simulink model "zad1"  (Simulink 7.7)
settings: Solver=ode45  StartTime=0.0  StopTime=t_sim  RelTol=1e-3
values from neighbouring files (symbols this model uses):
  ICX = -0.2    [zadatak1.m]    (also in zadatak2.m = 2; zadatak4.m = 0.4)
  ICY = -0.6    [zadatak1.m]    (also in zadatak2.m = 4; zadatak4.m = 1)
settings Model: Creator=Domagoj  LastModifiedBy=Domagoj
settings DebuggingCC: SolverPrmCheckMsg=none

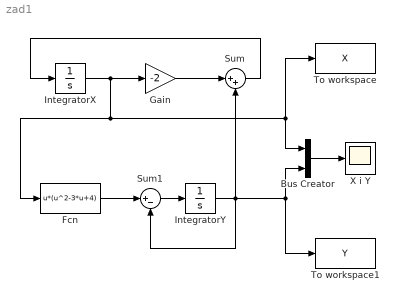
== system zad1 ==
  Bus Creator : BusCreator  Inputs=2
  Fcn : Fcn  Expr=u*(u^2-3*u+4)
  Gain : Gain  Gain=-2
  IntegratorX : Integrator  InitialCondition=ICX  UpperSaturationLimit=10000
  IntegratorY : Integrator  InitialCondition=ICY  UpperSaturationLimit=10000
  Sum : Sum  Inputs=|++
  Sum1 : Sum  Inputs=|+-
  To workspace : ToWorkspace  VariableName=X  SampleTime=-1  SaveFormat=Array
  To workspace1 : ToWorkspace  VariableName=Y  SampleTime=-1  SaveFormat=Array
  X i Y : Scope
      settings: SaveName=ScopeData2
  wires:
  Gain/1 -> Sum/1
  Sum/1 -> IntegratorX/1
  IntegratorX/1 -> Gain/1, To workspace/1, Bus Creator/1, Fcn/1
  IntegratorY/1 -> To workspace1/1, Bus Creator/2, Sum/2, Sum1/2
  Bus Creator/1 -> X i Y/1
  Sum1/1 -> IntegratorY/1
  Fcn/1 -> Sum1/1
